simulink subsystem "Actuator1"  (R2022a)
settings: Solver=VariableStepAuto  StartTime=0.0  StopTime=10.0  RelTol=1e-3
undefined symbols (not defined in the file or in its folder): actuator, room
libraries: fl_lib x10, ee_lib x6, SimscapeFluids_lib x2
settings Model: Creator=mmarq  LastModifiedBy=mmarq

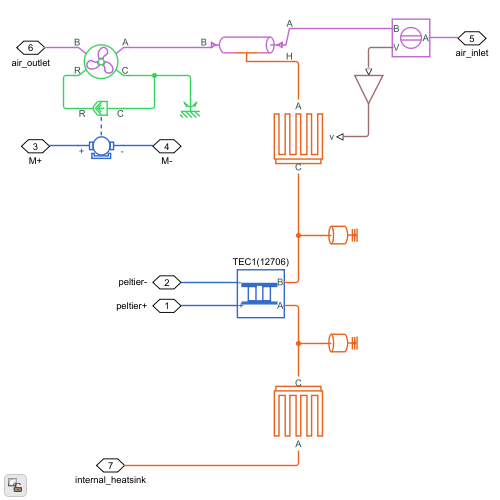
[thumbnail: Simulink's stored preview of the top-level diagram]
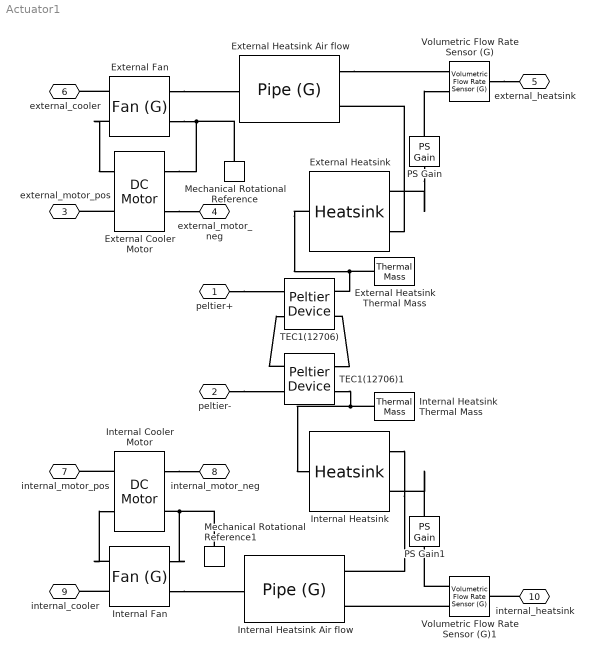
== system Actuator1 ==
  External Heatsink : ee_lib/Passive/Thermal/Heatsink  parameterization=ee.enum.passive.thermal.heatsinkParam.rectangularFin  convection=ee.enum.passive.thermal.heatsinkConvection.specifyFlowSpeed  T_vec_Q=[10, 30, 50, 70, 90] K  v_vec_Q=[0, 1, 2, 3] m/s  Q_TLU1=[6.1, 23.6, 44.5, 67.5, 92.3] W  Q_TLU2=[6.1, 18.8, 22.8, 25.7; 23.6, 61.1, 73, 81.5; 44.5, 106.4, 125.9, 140.1; 67.5, 153.5, 180.7, 200.3; 92.3, 202.1, 236.9, 262] W  T_vec_h=[10, 30, 50, 70, 90] K  v_vec_h=[0, 1, 2, 3] m/s  h_TLU1=[5.4, 7.02, 7.98, 8.68, 9.26] W/(K*m^2)  h_TLU2=[5.4, 17.86, 22.17, 25.41; 7.02, 19.49, 23.8, 27.03; 7.97, 20.44, 24.75, 27.99; 8.68, 21.15, 25.46, 28.69; 9.26, 21.73, 26.04, 29.27] W/(K*m^2)  h_vec=[5, 10, 15, 20, 25, 30] W/(K*m^2)  eff_TLU=[96.97, 94.16, 91.53, 89.08, 86.78, 84.62]  height=actuator.extHeatSink.fh m  thick=actuator.extHeatSink.ft m  depth=actuator.extHeatSink.fd m  gap=actuator.extHeatSink.fg m  num_fins=actuator.extHeatSink.fn  k_fin=actuator.extHeatSink.ftc W/(K*m)  A_total=0.1171 m^2  nu=1.51e-5 m^2/s  alpha=2.07e-5 m^2/s  k_fluid=25e-3 W/(K*m)  beta=3.3e-3 1/K  mass=0.35 kg  sp_heat=437 J/(K*kg)  T_hs_specify=on  T_hs_priority=High  T_hs=room.env_temp + 273 K  T_hs_nominal_specify=off  T_hs_nominal_unit=K  T_hs_nominal_value=1  Q_A_specify=off  Q_A_priority=None  Q_A=0 W  Q_A_nominal_specify=off  Q_A_nominal_unit=W  Q_A_nominal_value=1  Q_C_specify=off  Q_C_priority=None  Q_C=0 W  Q_C_nominal_specify=off  Q_C_nominal_unit=W  Q_C_nominal_value=1
      settings: SourceProductBaseCode=PS  InternalSimscapePortConfiguration="{\"Bottom\":[{\"id\":\"C\",\"label\":\"C\",\"type\":\"foundation.thermal.thermal\"}],\"Left\":[{\"id\":\"v\",\"label\":\"v\",\"type\":\"input\"}],\"Right\":[],\"Top\":[{\"id\":\"A\",\"label\":\"A\",\"type\":\"foundation.thermal.thermal\"}]}"
  External Cooler Motor : ee_lib/Electromechanical/Brushed Motors/DC Motor  field_option=ee.enum.field_option.pm  Rf=100 Ohm  Lf=1 H  Laf=0.15 H  If0=0 A  parameterization=ee.enum.dcparam_option.circuit_param  Ra=actuator.extDC.ra Ohm  La=actuator.extDC.la H  emf_or_torque=ee.enum.emf_or_torque.kv  Kv=actuator.extDC.kemf V/rpm  Ki=6.876e-4 N*m/A  T_stall=0.24e-3 N*m  w_max=actuator.extCooler.ref_cspeed*1.1 rpm  w_rated=actuator.extCooler.ref_cspeed rpm  P_rated=3.5 W  V_rated=12 V  lam_param=ee.enum.lam_param.damping  i_noload=0.29 A  V_i_noload=12 V  J=0.01 cm^2*g  lam=0 N*m*s/rad  speed0=0 rpm  enable_fault_armature=simscape.enum.onoff.off  rev_faulted=1 / 3  G_faulted_armature=1e-5 S  fault_trigger_armature=ee.enum.faults.faultTrigger.temporal  t_fault_armature=1 s  max_permissible_current_armature=inf A  t_fail_on_current_armature=1 s  enable_fault_field=simscape.enum.onoff.off  G_faulted_field=1e-5 S  fault_trigger_field=ee.enum.faults.faultTrigger.temporal  t_fault_field=1 s  max_permissible_current_field=inf A  t_fail_on_current_field=1 s  fault_action=simscape.enum.assert.action.none  alpha=3.93e-3 1/K  Tmeas=25 degC  thermal_mass=100 J/K  initial_temperature=25 degC
  External Fan : SimscapeFluids_lib/Gas/Turbomachinery/Fan (G)  fan_parameterization=fluids.gas.turbomachinery.enum.FanParameterization.Table1D  mechanical_power_spec=fluids.gas.turbomachinery.enum.FanMechanicalPowerSpec.Efficiency  flow_rate_nominal=0.12 m^3/s  pressure_nominal=5400 Pa  eta_nominal=0.40  power_nominal=1620 W  pressure_max=6400 Pa  flow_rate_max=0.24 m^3/s  omega_ref_nominal=3000 rpm  flow_rate_1D_TLU=actuator.extCooler.nominal_vfr_vec m^3/s  pressure_1D_TLU=actuator.extCooler.nominal_spg_vec Pa  eta_1D_TLU=actuator.extCooler.nominal_eff_vec  power_1D_TLU=[693, 900, 1107, 1267, 1363, 1452] W  omega_ref_1D=actuator.extCooler.ref_cspeed rpm  rho_ref_1D=1.2 kg/m^3  omega_dp_TLU=[2400; 3000; 3600] rpm  flow_rate_dp_TLU=[.0278, .0556, .0833, .111, .139, .167] m^3/s  pressure_dp_TLU=[4111, 4010, 3551, 2881, 2167, 1453; 6410, 6375, 6018, 5366, 4501, 3609; 9217, 9285, 9022, 8428, 7552, 6482] Pa  eta_dp_TLU=[.3, .434, .468, .459, .4, .3; .257, .394, .453, .47, .459, .415; .225, .359, .434, .461, .47, .459]  power_dp_TLU=[381, 514, 632, 697, 753, 809; 693, 900, 1107, 1267, 1363, 1452; 1139, 1438, 1732, 2029, 2233, 2358] W  rho_ref_dp=1.2 kg/m^3  omega_q_TLU=[2990; 3450; 3867] rpm  pressure_q_TLU=[31, 62, 93, 124] Pa  flow_rate_q_TLU=[.802, .759, .703, .611; .936, .902, .862, .81; 1.056, 1.027, .994, .956] m^3/s  eta_q_TLU=[.088, .162, .22, .261; .068, .128, .18, .222; .055, .105, .148, .188]  power_q_TLU=[283, 290, 297, 290; 427, 437, 445, 452; 595, 606, 625, 631] W  rho_ref_q=1.2 kg/m^3  diameter_ratio=1  mech_orientation=fluids.gas.turbomachinery.enum.FanMechanicalOrientation.Positive  area_A=actuator.extCooler.area m^2  area_B=actuator.extCooler.area m^2
      settings: SourceProductBaseCode=SH  InternalSimscapePortConfiguration="{\"Bottom\":[],\"Left\":[{\"id\":\"A\",\"label\":\"A\",\"type\":\"foundation.gas.gas\"},{\"id\":\"C\",\"label\":\"C\",\"type\":\"foundation.mechanical.rotational.rotational\"}],\"Right\":[{\"id\":\"B\",\"label\":\"B\",\"type\":\"foundation.gas.gas\"},{\"id\":\"R\",\"label\":\"R\",\"type\":\"foundation.mechanical.rotational.rotational\"}],\"Top\":[]}"
  External Heatsink Thermal Mass : fl_lib/Thermal/Thermal Elements/Thermal Mass  mass=actuator.extHeatSink.basemass kg  sp_heat=actuator.extHeatSink.specific_heat J/(K*kg)  T_specify=on  T_priority=High  T=room.env_temp + 273 K  T_nominal_specify=off  T_nominal_unit=K  T_nominal_value=1  Q_specify=off  Q_priority=None  Q=0 W  Q_nominal_specify=off  Q_nominal_unit=W  Q_nominal_value=1
      settings: SourceProductBaseCode=PW,SS,VE
  External Heatsink Air flow : fl_lib/Gas/Elements/Pipe (G)  length=actuator.extHeatSink.pl m  area=actuator.extHeatSink.pca m^2  Dh=actuator.extHeatSink.phd m  length_add=actuator.extHeatSink.pl m  roughness=15e-6 m  Re_lam=2000  Re_tur=4000  shape_factor=64  Nu_lam=3.66  p_I_specify=off  p_I_priority=High  p_I=0.101325 MPa  p_I_nominal_specify=off  p_I_nominal_unit=MPa  p_I_nominal_value=1  T_I_specify=on  T_I_priority=High  T_I=room.env_temp + 273 K  T_I_nominal_specify=off  T_I_nominal_unit=K  T_I_nominal_value=1  rho_pipe_specify=off  rho_pipe_priority=None  rho_pipe=1.2 kg/m^3  rho_pipe_nominal_specify=off  rho_pipe_nominal_unit=kg/m^3  rho_pipe_nominal_value=1
      settings: SourceProductBaseCode=PW,SS,VE
  Internal Heatsink : ee_lib/Passive/Thermal/Heatsink  parameterization=ee.enum.passive.thermal.heatsinkParam.rectangularFin  convection=ee.enum.passive.thermal.heatsinkConvection.specifyFlowSpeed  T_vec_Q=[10, 30, 50, 70, 90] K  v_vec_Q=[0, 1, 2, 3] m/s  Q_TLU1=[6.1, 23.6, 44.5, 67.5, 92.3] W  Q_TLU2=[6.1, 18.8, 22.8, 25.7; 23.6, 61.1, 73, 81.5; 44.5, 106.4, 125.9, 140.1; 67.5, 153.5, 180.7, 200.3; 92.3, 202.1, 236.9, 262] W  T_vec_h=[10, 30, 50, 70, 90] K  v_vec_h=[0, 1, 2, 3] m/s  h_TLU1=[5.4, 7.02, 7.98, 8.68, 9.26] W/(K*m^2)  h_TLU2=[5.4, 17.86, 22.17, 25.41; 7.02, 19.49, 23.8, 27.03; 7.97, 20.44, 24.75, 27.99; 8.68, 21.15, 25.46, 28.69; 9.26, 21.73, 26.04, 29.27] W/(K*m^2)  h_vec=[5, 10, 15, 20, 25, 30] W/(K*m^2)  eff_TLU=[96.97, 94.16, 91.53, 89.08, 86.78, 84.62]  height=actuator.intHeatSink.fh m  thick=actuator.intHeatSink.ft m  depth=actuator.intHeatSink.fd m  gap=actuator.intHeatSink.fg m  num_fins=actuator.intHeatSink.fn  k_fin=actuator.intHeatSink.ftc W/(K*m)  A_total=0.1171 m^2  nu=1.51e-5 m^2/s  alpha=2.07e-5 m^2/s  k_fluid=25e-3 W/(K*m)  beta=3.3e-3 1/K  mass=0.35 kg  sp_heat=437 J/(K*kg)  T_hs_specify=on  T_hs_priority=High  T_hs=room.env_temp + 273 K  T_hs_nominal_specify=off  T_hs_nominal_unit=K  T_hs_nominal_value=1  Q_A_specify=off  Q_A_priority=None  Q_A=0 W  Q_A_nominal_specify=off  Q_A_nominal_unit=W  Q_A_nominal_value=1  Q_C_specify=off  Q_C_priority=None  Q_C=0 W  Q_C_nominal_specify=off  Q_C_nominal_unit=W  Q_C_nominal_value=1
      settings: SourceProductBaseCode=PS  InternalSimscapePortConfiguration="{\"Bottom\":[{\"id\":\"C\",\"label\":\"C\",\"type\":\"foundation.thermal.thermal\"}],\"Left\":[{\"id\":\"v\",\"label\":\"v\",\"type\":\"input\"}],\"Right\":[],\"Top\":[{\"id\":\"A\",\"label\":\"A\",\"type\":\"foundation.thermal.thermal\"}]}"
  Internal Cooler Motor : ee_lib/Electromechanical/Brushed Motors/DC Motor  field_option=ee.enum.field_option.pm  Rf=100 Ohm  Lf=1 H  Laf=0.15 H  If0=0 A  parameterization=ee.enum.dcparam_option.circuit_param  Ra=actuator.intDC.ra Ohm  La=actuator.intDC.la H  emf_or_torque=ee.enum.emf_or_torque.kv  Kv=actuator.intDC.kemf V/rpm  Ki=6.876e-4 N*m/A  T_stall=0.24e-3 N*m  w_max=actuator.intCooler.ref_cspeed*1.1 rpm  w_rated=actuator.intCooler.ref_cspeed rpm  P_rated=0.72 W  V_rated=12 V  lam_param=ee.enum.lam_param.damping  i_noload=0.07 A  V_i_noload=12 V  J=0.01 cm^2*g  lam=0 N*m*s/rad  speed0=0 rpm  enable_fault_armature=simscape.enum.onoff.off  rev_faulted=1 / 3  G_faulted_armature=1e-5 S  fault_trigger_armature=ee.enum.faults.faultTrigger.temporal  t_fault_armature=1 s  max_permissible_current_armature=inf A  t_fail_on_current_armature=1 s  enable_fault_field=simscape.enum.onoff.off  G_faulted_field=1e-5 S  fault_trigger_field=ee.enum.faults.faultTrigger.temporal  t_fault_field=1 s  max_permissible_current_field=inf A  t_fail_on_current_field=1 s  fault_action=simscape.enum.assert.action.none  alpha=3.93e-3 1/K  Tmeas=25 degC  thermal_mass=100 J/K  initial_temperature=25 degC
  Internal Fan : SimscapeFluids_lib/Gas/Turbomachinery/Fan (G)  fan_parameterization=fluids.gas.turbomachinery.enum.FanParameterization.Table1D  mechanical_power_spec=fluids.gas.turbomachinery.enum.FanMechanicalPowerSpec.Efficiency  flow_rate_nominal=0.12 m^3/s  pressure_nominal=5400 Pa  eta_nominal=0.40  power_nominal=1620 W  pressure_max=6400 Pa  flow_rate_max=0.24 m^3/s  omega_ref_nominal=3000 rpm  flow_rate_1D_TLU=actuator.intCooler.nominal_vfr_vec m^3/s  pressure_1D_TLU=actuator.intCooler.nominal_spg_vec Pa  eta_1D_TLU=actuator.intCooler.nominal_eff_vec  power_1D_TLU=[693, 900, 1107, 1267, 1363, 1452] W  omega_ref_1D=actuator.intCooler.ref_cspeed rpm  rho_ref_1D=1.2 kg/m^3  omega_dp_TLU=[2400; 3000; 3600] rpm  flow_rate_dp_TLU=[.0278, .0556, .0833, .111, .139, .167] m^3/s  pressure_dp_TLU=[4111, 4010, 3551, 2881, 2167, 1453; 6410, 6375, 6018, 5366, 4501, 3609; 9217, 9285, 9022, 8428, 7552, 6482] Pa  eta_dp_TLU=[.3, .434, .468, .459, .4, .3; .257, .394, .453, .47, .459, .415; .225, .359, .434, .461, .47, .459]  power_dp_TLU=[381, 514, 632, 697, 753, 809; 693, 900, 1107, 1267, 1363, 1452; 1139, 1438, 1732, 2029, 2233, 2358] W  rho_ref_dp=1.2 kg/m^3  omega_q_TLU=omega_vec rpm  pressure_q_TLU=dp_vec Pa  flow_rate_q_TLU=flow_rate_TLU lpm  eta_q_TLU=ones(3,22).*0.3  power_q_TLU=[283, 290, 297, 290; 427, 437, 445, 452; 595, 606, 625, 631] W  rho_ref_q=1.2 kg/m^3  diameter_ratio=1  mech_orientation=fluids.gas.turbomachinery.enum.FanMechanicalOrientation.Positive  area_A=actuator.intCooler.area m^2  area_B=actuator.intCooler.area m^2
      settings: SourceProductBaseCode=SH  InternalSimscapePortConfiguration="{\"Bottom\":[],\"Left\":[{\"id\":\"A\",\"label\":\"A\",\"type\":\"foundation.gas.gas\"},{\"id\":\"C\",\"label\":\"C\",\"type\":\"foundation.mechanical.rotational.rotational\"}],\"Right\":[{\"id\":\"B\",\"label\":\"B\",\"type\":\"foundation.gas.gas\"},{\"id\":\"R\",\"label\":\"R\",\"type\":\"foundation.mechanical.rotational.rotational\"}],\"Top\":[]}"
  Internal Heatsink Thermal Mass : fl_lib/Thermal/Thermal Elements/Thermal Mass  mass=actuator.intHeatSink.basemass kg  sp_heat=actuator.intHeatSink.specific_heat J/(K*kg)  T_specify=on  T_priority=High  T=room.env_temp + 273 K  T_nominal_specify=off  T_nominal_unit=K  T_nominal_value=1  Q_specify=off  Q_priority=None  Q=0 W  Q_nominal_specify=off  Q_nominal_unit=W  Q_nominal_value=1
      settings: SourceProductBaseCode=PW,SS,VE
  Internal Heatsink Air flow : fl_lib/Gas/Elements/Pipe (G)  length=actuator.extHeatSink.pl m  area=actuator.extHeatSink.pca m^2  Dh=actuator.extHeatSink.phd m  length_add=actuator.extHeatSink.pl m  roughness=15e-6 m  Re_lam=2000  Re_tur=4000  shape_factor=64  Nu_lam=3.66  p_I_specify=off  p_I_priority=High  p_I=0.101325 MPa  p_I_nominal_specify=off  p_I_nominal_unit=MPa  p_I_nominal_value=1  T_I_specify=on  T_I_priority=High  T_I=room.env_temp + 273 K  T_I_nominal_specify=off  T_I_nominal_unit=K  T_I_nominal_value=1  rho_pipe_specify=off  rho_pipe_priority=None  rho_pipe=1.2 kg/m^3  rho_pipe_nominal_specify=off  rho_pipe_nominal_unit=kg/m^3  rho_pipe_nominal_value=1
      settings: SourceProductBaseCode=PW,SS,VE
  Mechanical Rotational Reference : fl_lib/Mechanical/Rotational Elements/Mechanical Rotational Reference
      settings: SourceProductBaseCode=PW,SS,VE
  Mechanical Rotational Reference1 : fl_lib/Mechanical/Rotational Elements/Mechanical Rotational Reference
      settings: SourceProductBaseCode=PW,SS,VE
  PS Gain : fl_lib/Physical Signals/Functions/PS Gain  gain=1/actuator.extHeatSink.pca m^-2
      settings: SourceProductBaseCode=PW,SS,VE
  PS Gain1 : fl_lib/Physical Signals/Functions/PS Gain  gain=1/actuator.extHeatSink.pca m^-2
      settings: SourceProductBaseCode=PW,SS,VE
  TEC1(12706) : ee_lib/Sensors & Transducers/Peltier Device  alpha=actuator.peltier.seebeck V/K  R=actuator.peltier.r Ohm  K=actuator.peltier.tc W/K
      settings: SourceProductBaseCode=PS  InternalSimscapePortConfiguration="{\"Bottom\":[],\"Left\":[{\"id\":\"p\",\"label\":\"+\",\"type\":\"foundation.electrical.electrical\"},{\"id\":\"n\",\"label\":\"-\",\"type\":\"foundation.electrical.electrical\"}],\"Right\":[{\"id\":\"A\",\"label\":\"A\",\"type\":\"foundation.thermal.thermal\"},{\"id\":\"B\",\"label\":\"B\",\"type\":\"foundation.thermal.thermal\"}],\"Top\":[]}"
  TEC1(12706)1 : ee_lib/Sensors & Transducers/Peltier Device  alpha=actuator.peltier.seebeck V/K  R=actuator.peltier.r Ohm  K=actuator.peltier.tc W/K
      settings: SourceProductBaseCode=PS  InternalSimscapePortConfiguration="{\"Bottom\":[],\"Left\":[{\"id\":\"p\",\"label\":\"+\",\"type\":\"foundation.electrical.electrical\"},{\"id\":\"n\",\"label\":\"-\",\"type\":\"foundation.electrical.electrical\"}],\"Right\":[{\"id\":\"A\",\"label\":\"A\",\"type\":\"foundation.thermal.thermal\"},{\"id\":\"B\",\"label\":\"B\",\"type\":\"foundation.thermal.thermal\"}],\"Top\":[]}"
  Volumetric Flow Rate Sensor (G) : fl_lib/Gas/Sensors/Volumetric Flow Rate Sensor (G)
      settings: SourceProductBaseCode=PW,SS,VE  InternalSimscapePortConfiguration="{\"Bottom\":[],\"Left\":[{\"id\":\"A\",\"label\":\"A\",\"type\":\"foundation.gas.gas\"}],\"Right\":[{\"id\":\"B\",\"label\":\"B\",\"type\":\"foundation.gas.gas\"},{\"id\":\"V\",\"label\":\"V\",\"type\":\"output\"}],\"Top\":[]}"
  Volumetric Flow Rate Sensor (G)1 : fl_lib/Gas/Sensors/Volumetric Flow Rate Sensor (G)
      settings: SourceProductBaseCode=PW,SS,VE  InternalSimscapePortConfiguration="{\"Bottom\":[],\"Left\":[{\"id\":\"A\",\"label\":\"A\",\"type\":\"foundation.gas.gas\"}],\"Right\":[{\"id\":\"B\",\"label\":\"B\",\"type\":\"foundation.gas.gas\"},{\"id\":\"V\",\"label\":\"V\",\"type\":\"output\"}],\"Top\":[]}"
  peltier+ : PMIOPort  Side=Left
  peltier- : PMIOPort  Port=2  Side=Left
  external_motor_pos : PMIOPort  Port=3  Side=Left
  external_motor_neg : PMIOPort  Port=4  Side=Left
  external_heatsink : PMIOPort  Port=5  Side=Left
  external_cooler : PMIOPort  Port=6  Side=Left
  internal_motor_pos : PMIOPort  Port=7  Side=Left
  internal_motor_neg : PMIOPort  Port=8  Side=Left
  internal_cooler : PMIOPort  Port=9  Side=Left
  internal_heatsink : PMIOPort  Port=10  Side=Left
  connections:
  TEC1(12706)/RConn2 -- External Heatsink/RConn1 -- External Heatsink Thermal Mass/LConn1
  External Cooler Motor/RConn2 -- External Fan/LConn2 -- Mechanical Rotational Reference/LConn1
  TEC1(12706)1/RConn1 -- Internal Heatsink/RConn1 -- Internal Heatsink Thermal Mass/LConn1
  Internal Fan/LConn2 -- Internal Cooler Motor/RConn2 -- Mechanical Rotational Reference1/LConn1
  External Heatsink Air flow/LConn1 -- Volumetric Flow Rate Sensor (G)/RConn1
  External Fan/LConn1 -- External Heatsink Air flow/RConn1
  External Fan/RConn2 -- External Cooler Motor/LConn2
  External Heatsink/LConn2 -- External Heatsink Air flow/LConn2
  PS Gain/RConn1 -- External Heatsink/LConn1
  PS Gain/LConn1 -- Volumetric Flow Rate Sensor (G)/RConn2
  External Cooler Motor/LConn1 -- external_motor_pos/RConn1
  External Fan/RConn1 -- external_cooler/RConn1
  External Cooler Motor/RConn1 -- external_motor_neg/RConn1
  Volumetric Flow Rate Sensor (G)/LConn1 -- external_heatsink/RConn1
  TEC1(12706)1/LConn2 -- TEC1(12706)/LConn1
  TEC1(12706)1/RConn2 -- TEC1(12706)/RConn1
  Internal Cooler Motor/RConn1 -- internal_motor_neg/RConn1
  Internal Cooler Motor/LConn1 -- internal_motor_pos/RConn1
  Internal Fan/RConn1 -- internal_cooler/RConn1
  Internal Fan/RConn2 -- Internal Cooler Motor/LConn2
  Internal Fan/LConn1 -- Internal Heatsink Air flow/RConn1
  Internal Heatsink/LConn2 -- Internal Heatsink Air flow/LConn2
  PS Gain1/RConn1 -- Internal Heatsink/LConn1
  Volumetric Flow Rate Sensor (G)1/RConn1 -- Internal Heatsink Air flow/LConn1
  Volumetric Flow Rate Sensor (G)1/RConn2 -- PS Gain1/LConn1
  internal_heatsink/RConn1 -- Volumetric Flow Rate Sensor (G)1/LConn1
  peltier+/RConn1 -- TEC1(12706)/LConn2
  peltier-/RConn1 -- TEC1(12706)1/LConn1
